simulink model "ampc_cstr_linearization_modified"  (R2022b)
settings: Solver=ode45  StartTime=0  StopTime=48  MaxStep=0.5*Ts  RelTol=1e-3  EnableMultiTasking=on
undefined symbols (not defined in the file): Np, Nu, qu, qy, Ts, u0, umax, umin, x0
libraries: mpclib x1, simulink x1
settings Model: Creator=The MathWorks, Inc.  LastModifiedBy=ZacksZephyrusM16
settings SolverCC: AlgebraicLoopSolver=TrustRegion
settings DataIOCC: ExternalInput=ExtIn  InitialState=[311.267; 8.5695]  SaveFormat=Structure  SaveOutput=off  SignalLogging=off  SaveTime=off  ReturnWorkspaceOutputs=off  SignalLoggingName=logsOut
settings OptimizationCC: BooleanDataType=off  DefaultParameterBehavior=Inlined  InlineInvariantSignals=on  BufferReuse=off  ExpressionDepthLimit=2147483647  InitFltsAndDblsToZero=on  LifeSpan=inf
settings DebuggingCC: SaveWithParameterizedLinksMsg=none  UnderspecifiedInitializationDetection=Classic  MergeDetectMultiDrivingBlocksExec=none  CheckExecutionContextPreStartOutputMsg=on  SignalResolutionControl=TryResolveAllWithWarning  MultiTaskDSMMsg=warning  MultiTaskCondExecSysMsg=none  UnconnectedInputMsg=warning  UnconnectedOutputMsg=warning  UnconnectedLineMsg=warning  StateNameClashWarn=warning  SFUnexpectedBacktrackingDiag=warning  SFNoUnconditionalDefaultTransitionDiag=warning  SFExecutionAtInitializationDiag=none  SFMachineParentedDataDiag=warning  ArithmeticOperatorsInVariantConditions=warning
settings HardwareCC: ProdBitPerPointer=32  ProdBitPerSizeT=32  ProdBitPerPtrDiffT=32  ProdLargestAtomicFloat=None  ProdIntDivRoundTo=Undefined  ProdEndianess=Unspecified  ProdWordSize=32  ProdHWDeviceType=32-bit Generic  TargetBitPerPointer=64  TargetBitPerSizeT=64  TargetBitPerPtrDiffT=64  TargetLongLongMode=on  TargetIntDivRoundTo=Zero  TargetEndianess=LittleEndian  TargetWordSize=64  TargetHWDeviceType=MATLAB Host  ProdEqTarget=off
settings ModelReferenceCC: EnableRefExpFcnMdlSchedulingChecks=on  PropagateSignalLabelsOutOfModel=off
settings SFSimCC: SimUseLocalCustomCode=off  CustomCodeUndefinedFunction=UseInterfaceOnly
settings RTWCC: RTWUseLocalCustomCode=off  DLArmComputeVersion=19.05
settings CodeAppCC: StateflowObjectComments=on
settings GRTTargetCC: TargetFcnLib=ansi_tfl_tmw.mat  TargetLangStandard=C89/C90 (ANSI)  CombineOutputUpdateFcns=off  GRTInterface=on
settings ConfigComp: CovMetricSettings=dw  CovSaveCumulativeToWorkspaceVar=on  CovSaveSingleToWorkspaceVar=on  CovExternalEMLEnable=off  CovSFcnEnable=off

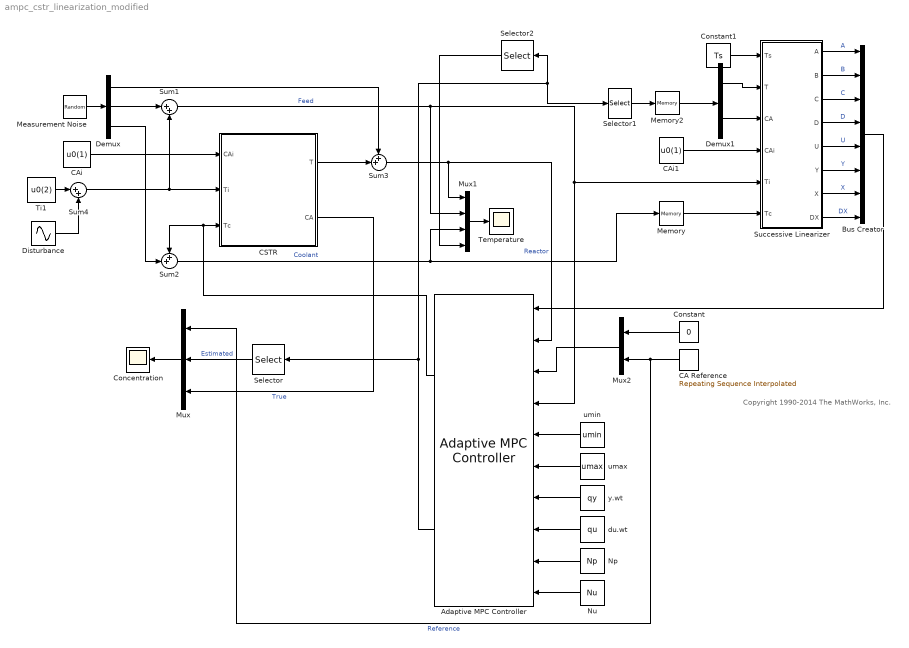
== system ampc_cstr_linearization_modified ==
  note: Copyright 1990-2014 The MathWorks, Inc.
  Adaptive MPC Controller : mpclib/Adaptive MPC Controller  SCDEnableBlockLinearizationSpecification=on  mpcobj=mpcobj  enable_value=0  updateMPCinCallerWorkspace=on  md_inport=on  mv_inport=off  uref_inport=off  return_cost=off  return_mvseq=off  return_qpstatus=off  return_xseq=off  return_state=on  return_ovseq=off  state_inport=off  isltv_plant=off  umin_inport=on  umax_inport=on  ymin_inport=off  ymax_inport=off  cc_inport=off  ywt_inport=on  uwt_inport=off  duwt_inport=on  rhoeps_inport=off  pm_inport=on  MaximumP=40  HorizonChoice=VariableHorizon  BlockDataType=double  SampleTimeInherited=off  switch_inport=off
  Bus Creator : BusCreator  Inputs=8
  CA Reference : simulink/Sources/Repeating Sequence Interpolated  OutValues=[2, 2, 2, 2]  TimeValues="[0 50  150 200]"  LookUpMeth=Interpolation-Use End Values  tsamp=Ts  OutMin=[]  OutMax=[]  OutDataTypeStr=double  OutputDataTypeScalingMode=double  OutDataType=fixdt(0,8)  OutScaling=2^-10
  CAi : Constant  Value=u0(1)
  CAi1 : Constant  Value=u0(1)
  CSTR : Subsystem
  Concentration : Scope
  Constant : Constant  Value=0
  Constant1 : Constant  Value=Ts
  Demux : Demux  Outputs=3
  Demux1 : Demux  Outputs=2
  Disturbance : Sin  Amplitude=2  Frequency=0.05  SampleTime=0
  Measurement Noise : RandomNumber  Mean=[0 0 0]  Variance=0.001*[1 1 1]  Seed=98325  SampleTime=Ts/5
  Memory : Memory  InitialCondition=u0(3)
  Memory2 : Memory  InitialCondition=x0
  Mux : Mux  Inputs=3
  Mux1 : Mux
  Mux2 : Mux  Inputs=2
  Np : Constant  Value=Np
  Nu : Constant  Value=Nu
  Selector : Selector  InputPortWidth=3  IndexOptions=Index vector (dialog)  Indices=[2]  OutputSizes=1
  Selector1 : Selector  InputPortWidth=3  IndexOptions=Index vector (dialog)  Indices=1:2  OutputSizes=1
  Selector2 : Selector  InputPortWidth=3  IndexOptions=Index vector (dialog)  Indices=1  OutputSizes=1
  Successive Linearizer : MATLAB Function  TreatAsAtomicUnit=on  SystemSampleTime=Ts
  Sum1 : Sum  Inputs=|++  SampleTime=Ts/5
  Sum2 : Sum  Inputs=++|  SampleTime=Ts/5
  Sum3 : Sum  Inputs=++|  SampleTime=Ts/5
  Sum4 : Sum  Inputs=|++  SampleTime=Ts/5
  Temperature : Scope
  Ti1 : Constant  Value=u0(2)
  du.wt : Constant  Value=qu
  umax : Constant  Value=umax
  umin : Constant  Value=umin
  y.wt : Constant  Value=qy
  wires:
  CA Reference/1 -> Mux/1, Mux2/2  "Reference"
  Mux/1 -> Concentration/1
  Mux1/1 -> Temperature/1
  Sum1/1 -> Mux1/2, Adaptive MPC Controller/4, Successive Linearizer/5(Ti)  "Feed"
  Bus Creator/1 -> Adaptive MPC Controller/1
  Mux2/1 -> Adaptive MPC Controller/3
  CAi/1 -> CSTR/1(CAi)
  Measurement Noise/1 -> Demux/1
  Demux/1 -> Sum3/1
  Demux/2 -> Sum1/1
  Demux/3 -> Sum2/2
  Sum2/1 -> Mux1/3, Memory/1  "Coolant"
  Constant/1 -> Mux2/1
  Sum3/1 -> Adaptive MPC Controller/2, Mux1/1  "Reactor"
  CSTR/2(CA) -> Mux/3  "True"
  CSTR/1(T) -> Sum3/2
  Adaptive MPC Controller/1 -> Sum2/1, CSTR/3(Tc)
  Selector/1 -> Mux/2  "Estimated"
  Sum4/1 -> Sum1/2, CSTR/2(Ti)
  Successive Linearizer/1(A) -> Bus Creator/1  "A"
  Successive Linearizer/2(B) -> Bus Creator/2  "B"
  Successive Linearizer/3(C) -> Bus Creator/3  "C"
  Successive Linearizer/4(D) -> Bus Creator/4  "D"
  Successive Linearizer/5(U) -> Bus Creator/5  "U"
  Successive Linearizer/6(Y) -> Bus Creator/6  "Y"
  Successive Linearizer/7(X) -> Bus Creator/7  "X"
  Successive Linearizer/8(DX) -> Bus Creator/8  "DX"
  Demux1/1 -> Successive Linearizer/2(T)
  Demux1/2 -> Successive Linearizer/3(CA)
  Memory/1 -> Successive Linearizer/6(Tc)
  Memory2/1 -> Demux1/1
  Selector1/1 -> Memory2/1
  Adaptive MPC Controller/2 -> Selector2/1, Selector1/1, Selector/1
  CAi1/1 -> Successive Linearizer/4(CAi)
  umin/1 -> Adaptive MPC Controller/5
  umax/1 -> Adaptive MPC Controller/6
  y.wt/1 -> Adaptive MPC Controller/7
  du.wt/1 -> Adaptive MPC Controller/8
  Np/1 -> Adaptive MPC Controller/9
  Nu/1 -> Adaptive MPC Controller/10
  Constant1/1 -> Successive Linearizer/1(Ts)
  Disturbance/1 -> Sum4/2
  Ti1/1 -> Sum4/1
  Selector2/1 -> Mux1/4

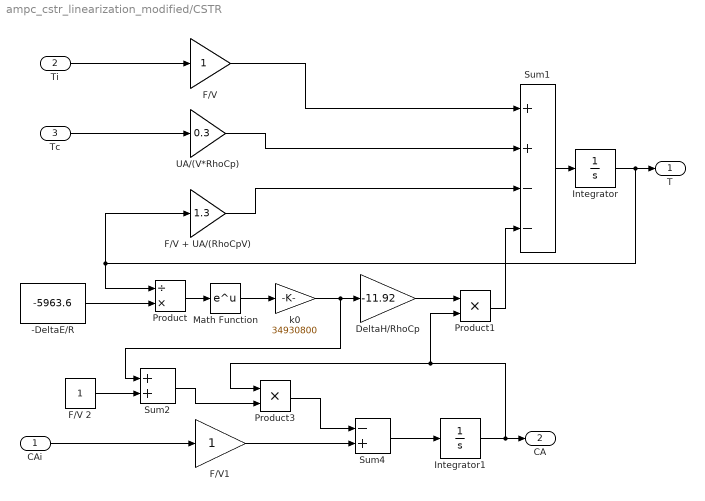
== system ampc_cstr_linearization_modified/CSTR ==
  CAi : Inport
  Ti : Inport  Port=2
  Tc : Inport  Port=3
  -DeltaE/R : Constant  Value=-5963.6
  DeltaH/RhoCp : Gain  Gain=-11.92  SaturateOnIntegerOverflow=on  OutDataTypeStr=Inherit: Same as input  ParamDataTypeStr=Inherit: Same as input
  F/V : Gain  SaturateOnIntegerOverflow=on  OutDataTypeStr=Inherit: Same as input  ParamDataTypeStr=Inherit: Same as input
  F/V + UA/(RhoCpV) : Gain  Gain=1.3  SaturateOnIntegerOverflow=on  OutDataTypeStr=Inherit: Same as input  ParamDataTypeStr=Inherit: Same as input
  F/V 2 : Constant
  F/V1 : Gain  SaturateOnIntegerOverflow=on  OutDataTypeStr=Inherit: Same as input  ParamDataTypeStr=Inherit: Same as input
  Integrator : Integrator  InitialCondition=311.2639  LimitOutput=on  LowerSaturationLimit=0
  Integrator1 : Integrator  InitialCondition=8.5698  LimitOutput=on  LowerSaturationLimit=0
  Math Function : Math  SignedPower=on
  Product : Product  Inputs=/*  InputSameDT=on  RndMeth=Zero  SaturateOnIntegerOverflow=on  OutDataTypeStr=Inherit: Same as first input
  Product1 : Product  InputSameDT=on  RndMeth=Zero  SaturateOnIntegerOverflow=on  OutDataTypeStr=Inherit: Same as first input
  Product3 : Product  InputSameDT=on  RndMeth=Zero  SaturateOnIntegerOverflow=on  OutDataTypeStr=Inherit: Same as first input
  Sum1 : Sum  Inputs=++--  InputSameDT=on  SaturateOnIntegerOverflow=on  OutDataTypeStr=Inherit: Same as first input
  Sum2 : Sum  InputSameDT=on  SaturateOnIntegerOverflow=on  OutDataTypeStr=Inherit: Same as first input
  Sum4 : Sum  Inputs=-+  InputSameDT=on  SaturateOnIntegerOverflow=on  OutDataTypeStr=Inherit: Same as first input
  UA/(V*RhoCp) : Gain  Gain=0.3  SaturateOnIntegerOverflow=on  OutDataTypeStr=Inherit: Same as input  ParamDataTypeStr=Inherit: Same as input
  k0 : Gain  Gain=34930800  SaturateOnIntegerOverflow=on  OutDataTypeStr=Inherit: Same as input  ParamDataTypeStr=Inherit: Same as input
  T : Outport
  CA : Outport  Port=2
  wires:
  Sum2/1 -> Product3/2
  Tc/1 -> UA/(V*RhoCp)/1
  CAi/1 -> F/V1/1
  Ti/1 -> F/V/1
  F/V1/1 -> Sum4/2
  F/V 2/1 -> Sum2/2
  Integrator1/1 -> CA/1, Product3/1, Product1/2
  Sum4/1 -> Integrator1/1
  Product3/1 -> Sum4/1
  -DeltaE/R/1 -> Product/2
  k0/1 -> Sum2/1, DeltaH/RhoCp/1
  Product1/1 -> Sum1/4
  DeltaH/RhoCp/1 -> Product1/1
  Math Function/1 -> k0/1
  Product/1 -> Math Function/1
  F/V + UA/(RhoCpV)/1 -> Sum1/3
  UA/(V*RhoCp)/1 -> Sum1/2
  Integrator/1 -> T/1, F/V + UA/(RhoCpV)/1, Product/1
  Sum1/1 -> Integrator/1
  F/V/1 -> Sum1/1

== matlab function ampc_cstr_linearization_modified/Successive Linearizer ==
  data: Ts input; A output size=[2,2]; T input; B output size=[2,2]; CA input; CAi input; Ti input; Tc input; C output size=[2,2]; D output size=[2,2]; U output size=[2,1]; Y output size=[2,1]; X output size=[2,1]; DX output size=[2,1]
function [A, B, C, D, U, Y, X, DX] = fcn(Ts, T, CA, CAi, Ti, Tc)
%#codegen

% Define constant outputs
C = eye(2);
D = zeros(2,2);
% Nominal U are obtained from measurements
U = [Ti; Tc];
% Nominal X and Y are obtained from estimated MPC states
Y = [T; CA];
X = [T; CA];
% Analytical linearization of mechanistic CSTR model (continuous time)
[A, Bo] = getContinuous(T, CA, CAi, Ti, Tc);
% Convert continuous to discrete time
[A, Bo] = adasblocks_utilDicretizeModel(A, Bo, Ts);
% Last column of B contains the constant offset contribution.
DX = Bo(:,3);
B = Bo(:,1:2);

function [a, b] = getContinuous(T, CA, CAi, Ti, Tc)
% Define linear continuous-time matrices A and B for CSTR.  Last input is
% offset.

% Parameters
EaOverR = 5963.6;
lnA0 = 17.3689;
FoV = 1;                    % F/V [=] 1/s
A0 = exp(lnA0);             % Arrhenius pre-exponential, [=] 1/s
EoR = EaOverR;              % Ea/R [=] K
dHrCon = -11.92;            % delH/(Rho*C) [=] K-m3/kmol
UACon = 0.3;                % UA/(Rho*C*V) [=] 1/s
k = -A0*exp(-EoR/T);        % k is for rate of A production [=] 1/s
rA = k*CA;
% Nonlinear model time derivatives
dxdt = zeros(2,1);
dxdt(1) = (CAi - CA)*FoV + rA;
dxdt(2) = (Ti - T)*FoV + UACon*(Tc -T) + dHrCon*rA;
% Reaction rate partial derivatives
drAdCA = k;
drAdT = CA*k*EoR/(T^2);
% Continuous-time matrix: A
a = [(drAdCA - FoV)   drAdT
     dHrCon*drAdCA    (dHrCon*drAdT - FoV - UACon)];
% Continuous-time matrix: B
b = [0      0       dxdt(1)
     FoV    UACon   dxdt(2)];
% Make state indices consistent with x1 = T, x2 = CA
ix = [2,1];
a = a(ix,ix);
b = b(ix,:);
